simulink model "dev_RigTestWithNetwork"  (R2020b)
settings: Solver=VariableStepAuto  StartTime=0.0  StopTime=800  RelTol=1e-3
model workspace (MAT data in the model file):
  G_sup_tsp = Simulink.Signal
  G_sup_tsp.DataType = 'double'
  G_sup_tsp.Dimensions = -1
  G_sup_tsp.DimensionsMode = 'auto'
  G_sup_tsp.Complexity = 'real'
  G_sup_tsp.SampleTime = -1
  G_sup_tsp.SamplingMode = 'auto'
  G_sup_tsp.InitialValue = '175'
undefined symbols (not defined in the file): WLAN
libraries: truetime x9, IMT_Library x8, simulink_extras x4, slpidlib x2
settings Model: Creator=Mr_Li  LastModifiedBy=Mr_Li

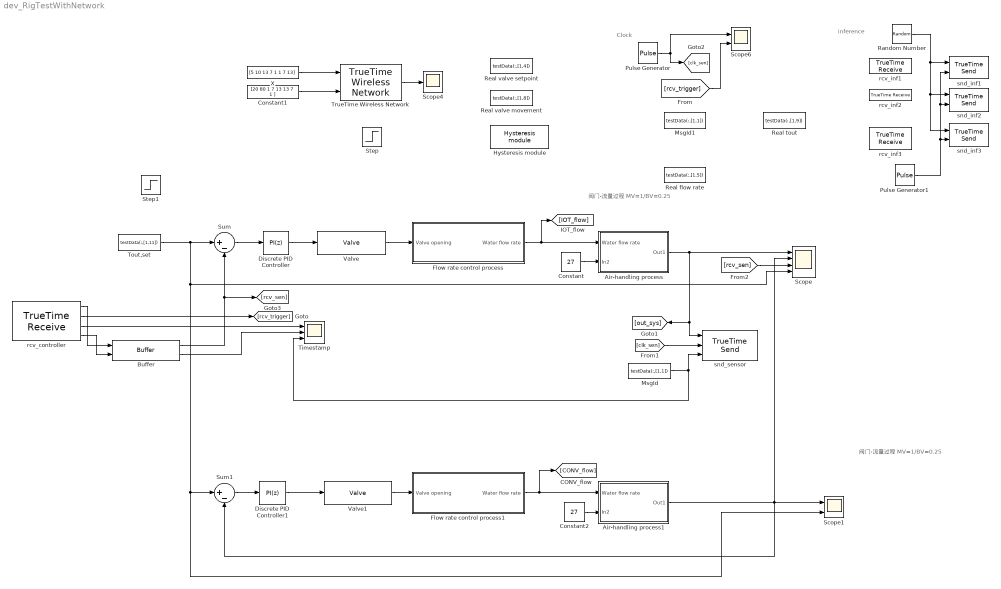
== system dev_RigTestWithNetwork ==
  note: inference
  note: 阀门-流量过程
      | MV=1/BV=0.25
  note: Clock
  note: 阀门-流量过程
      | MV=1/BV=0.25
  Air-handling process : Subsystem
  Air-handling process1 : Subsystem
  Buffer : IMT_Library/Buffer  initId=0  initValue=26
      settings: SourceProductName=Imitation
  Constant : Constant  Value=27
  Constant1 : Constant  Value=[20 80 1 7 13 13 7 1 ]  VectorParams1D=off
  Constant2 : Constant  Value=27
  Discrete PID Controller : slpidlib/PID Controller  Controller=PI  Form=Parallel  TimeDomain=Discrete-time  UseExternalTs=off  SampleTime=1  IntegratorMethod=Forward Euler  FilterMethod=Forward Euler  ControllerParametersSource=internal  P=0.5  I=0.0075  D=0  UseFilter=on  N=100  TunerSelectOption=Frequency Response Based  InitialConditionSource=internal  InitialConditionForIntegrator=0  InitialConditionForFilter=0  DifferentiatorICPrevScaledInput=0  ExternalReset=none  TrackingMode=off  Kt=1  LimitOutput=off  SatLimitsSource=internal  UpperSaturationLimit=inf  LowerSaturationLimit=-inf  LinearizeAsGain=off  AntiWindupMode=none  Kb=1  POutMin=[]  POutMax=[]  IOutMin=[]  IOutMax=[]  DOutMin=[]  DOutMax=[]  NOutMin=[]  NOutMax=[]  SumOutMin=[]  SumOutMax=[]  SaturationOutMin=[]  SaturationOutMax=[]  PParamMin=[]  PParamMax=[]  IParamMin=[]  IParamMax=[]  DParamMin=[]  DParamMax=[]  NParamMin=[]  NParamMax=[]  KbParamMin=[]  KbParamMax=[]  KtParamMin=[]  KtParamMax=[]  KbOutMin=[]  KbOutMax=[]  KtOutMin=[]  KtOutMax=[]  IntegratorOutMin=[]  IntegratorOutMax=[]  FilterOutMin=[]  FilterOutMax=[]  SumI1OutMin=[]  SumI1OutMax=[]  SumI2OutMin=[]  SumI2OutMax=[]  SumI3OutMin=[]  SumI3OutMax=[]  SumI4OutMin=[]  SumI4OutMax=[]  SumDOutMin=[]  SumDOutMax=[]  DifferentiatorOutMin=[]  DifferentiatorOutMax=[]  FilterDiffOutCoefMin=[]  FilterDiffOutCoefMax=[]  ReciprocalOutMin=[]  ReciprocalOutMax=[]  SumDenOutMin=[]  SumDenOutMax=[]  SumNumOutMin=[]  SumNumOutMax=[]  DivideOutMin=[]  DivideOutMax=[]  UdiffTsProdOutMin=[]  UdiffTsProdOutMax=[]  NTsProdOutMin=[]  NTsProdOutMax=[]  UintegralTsProdOutMin=[]  UintegralTsProdOutMax=[]  UngainTsProdOutMin=[]  UngainTsProdOutMax=[]  IntegratorContinuousStateAttributes=''  IntegratorStateMustResolveToSignalObject=off  IntegratorRTWStateStorageClass=Auto  FilterContinuousStateAttributes=''  FilterStateMustResolveToSignalObject=off  FilterRTWStateStorageClass=Auto  ParallelPVariant=InternalParameters  IdealPVariant=Disabled  IVariant=InternalParameters  DVariant=Disabled  IntegratorVariant=Discrete  SatVariant=Disabled  AWVariant=Passthrough  PCopyVariant=Disabled  TRVariant=Disabled  FdbkBlocksVariant=Forward  IdealPFdbkVariant=Disabled  SatFdbkVariant=Disabled  DerivativeFilterVariant=Disabled  NVariant=Disabled  NCopyVariant=Disabled_SignalSpec  FilterICVariant=Disabled  IntegratorICVariant=InternalICs  ExternalResetVariant=Disabled  TRSumVariant=Passthrough  SumFdbkVariant=Disabled  SumVariant=Sum_PI  TsampFilterVariant=InternalTs  TsampNgainVariant=Passthrough  TsampIntegralVariant=Passthrough  ExternalSaturationOutDataTypeStr=Inherit: Same as second input
  Discrete PID Controller1 : slpidlib/PID Controller  Controller=PI  Form=Parallel  TimeDomain=Discrete-time  UseExternalTs=off  SampleTime=1  IntegratorMethod=Forward Euler  FilterMethod=Forward Euler  ControllerParametersSource=internal  P=0.5  I=0.0075  D=0  UseFilter=on  N=100  TunerSelectOption=Frequency Response Based  InitialConditionSource=internal  InitialConditionForIntegrator=0  InitialConditionForFilter=0  DifferentiatorICPrevScaledInput=0  ExternalReset=none  TrackingMode=off  Kt=1  LimitOutput=off  SatLimitsSource=internal  UpperSaturationLimit=inf  LowerSaturationLimit=-inf  LinearizeAsGain=off  AntiWindupMode=none  Kb=1  POutMin=[]  POutMax=[]  IOutMin=[]  IOutMax=[]  DOutMin=[]  DOutMax=[]  NOutMin=[]  NOutMax=[]  SumOutMin=[]  SumOutMax=[]  SaturationOutMin=[]  SaturationOutMax=[]  PParamMin=[]  PParamMax=[]  IParamMin=[]  IParamMax=[]  DParamMin=[]  DParamMax=[]  NParamMin=[]  NParamMax=[]  KbParamMin=[]  KbParamMax=[]  KtParamMin=[]  KtParamMax=[]  KbOutMin=[]  KbOutMax=[]  KtOutMin=[]  KtOutMax=[]  IntegratorOutMin=[]  IntegratorOutMax=[]  FilterOutMin=[]  FilterOutMax=[]  SumI1OutMin=[]  SumI1OutMax=[]  SumI2OutMin=[]  SumI2OutMax=[]  SumI3OutMin=[]  SumI3OutMax=[]  SumI4OutMin=[]  SumI4OutMax=[]  SumDOutMin=[]  SumDOutMax=[]  DifferentiatorOutMin=[]  DifferentiatorOutMax=[]  FilterDiffOutCoefMin=[]  FilterDiffOutCoefMax=[]  ReciprocalOutMin=[]  ReciprocalOutMax=[]  SumDenOutMin=[]  SumDenOutMax=[]  SumNumOutMin=[]  SumNumOutMax=[]  DivideOutMin=[]  DivideOutMax=[]  UdiffTsProdOutMin=[]  UdiffTsProdOutMax=[]  NTsProdOutMin=[]  NTsProdOutMax=[]  UintegralTsProdOutMin=[]  UintegralTsProdOutMax=[]  UngainTsProdOutMin=[]  UngainTsProdOutMax=[]  IntegratorContinuousStateAttributes=''  IntegratorStateMustResolveToSignalObject=off  IntegratorRTWStateStorageClass=Auto  FilterContinuousStateAttributes=''  FilterStateMustResolveToSignalObject=off  FilterRTWStateStorageClass=Auto  ParallelPVariant=InternalParameters  IdealPVariant=Disabled  IVariant=InternalParameters  DVariant=Disabled  IntegratorVariant=Discrete  SatVariant=Disabled  AWVariant=Passthrough  PCopyVariant=Disabled  TRVariant=Disabled  FdbkBlocksVariant=Forward  IdealPFdbkVariant=Disabled  SatFdbkVariant=Disabled  DerivativeFilterVariant=Disabled  NVariant=Disabled  NCopyVariant=Disabled_SignalSpec  FilterICVariant=Disabled  IntegratorICVariant=InternalICs  ExternalResetVariant=Disabled  TRSumVariant=Passthrough  SumFdbkVariant=Disabled  SumVariant=Sum_PI  TsampFilterVariant=InternalTs  TsampNgainVariant=Passthrough  TsampIntegralVariant=Passthrough  ExternalSaturationOutDataTypeStr=Inherit: Same as second input
  Flow rate control process : Subsystem
  Flow rate control process1 : Subsystem
  Hysteresis module : IMT_Library/Hysteresis module  hysteresisSize=4.5
      settings: SourceProductName=Imitation
  MsgId : FromWorkspace  VariableName=testData(:,[1,1])  SampleTime=1
  MsgId1 : FromWorkspace  VariableName=testData(:,[1,1])  SampleTime=1
  Pulse Generator : DiscretePulseGenerator  SampleTime=0.5
  Pulse Generator1 : DiscretePulseGenerator
  Random Number : RandomNumber  SampleTime=1
  Real flow rate : FromWorkspace  VariableName=testData(:,[1,5])
  Real tout : FromWorkspace  VariableName=testData(:,[1,9])
  Real valve movement : FromWorkspace  VariableName=testData(:,[1,8])  SampleTime=1
  Real valve setpoint : FromWorkspace  VariableName=testData(:,[1,4])  SampleTime=1
  Scope : Scope  NumInputPorts=4
  Scope1 : Scope  NumInputPorts=2
  Scope4 : Scope
  Scope6 : Scope  NumInputPorts=2
  Step : Step  Time=18  After=0.31  SampleTime=0
  Step1 : Step  After=45  SampleTime=0
  Sum : Sum  Inputs=|+-
  Sum1 : Sum  Inputs=|+-
  Timestamp : Scope  NumInputPorts=3
  Tout,set : FromWorkspace  VariableName=testData(:,[1,11])  SampleTime=1
  TrueTime Wireless Network : truetime/TrueTime Wireless  Network  nwtype=802.11b (WLAN)  nwnbr=1  nnodes=8  rate=800000  minsize=272  transpower=30  threshold=-48  use_pathloss_function=default  pathloss=4.0  acktimeout=1  retrylimit=3  error_threshold=0.04  lossprob=0.4  seed=0  scheduleoutput=on  poweroutput=off
  Valve : IMT_Library/Valve  upper=101  lower=1.2  movementThreshold=1
      settings: SourceProductName=Imitation
  Valve1 : IMT_Library/Valve  upper=101  lower=1.2  movementThreshold=1
      settings: SourceProductName=Imitation
  X : Constant  Value="[5 10 13 7 1  1 7 13]"  VectorParams1D=off
  rcv_controller : truetime/TrueTime Receive  nwnbr=1  receiver=2  outdim=1  triggeroutput=on  senderoutput=off  lengthoutput=off  priorityoutput=off  timestampoutput=on  signalpoweroutput=off  msgIDoutput=on
  rcv_inf1 : truetime/TrueTime Receive  nwnbr=1  receiver=4  outdim=1  triggeroutput=off  senderoutput=off  lengthoutput=off  priorityoutput=off  timestampoutput=off  signalpoweroutput=off  msgIDoutput=off
  rcv_inf2 : truetime/TrueTime Receive  nwnbr=1  receiver=6  outdim=1  triggeroutput=off  senderoutput=off  lengthoutput=off  priorityoutput=off  timestampoutput=off  signalpoweroutput=off  msgIDoutput=off
  rcv_inf3 : truetime/TrueTime Receive  nwnbr=1  receiver=8  outdim=1  triggeroutput=on  senderoutput=off  lengthoutput=off  priorityoutput=off  timestampoutput=off  signalpoweroutput=off  msgIDoutput=off
  snd_inf1 : truetime/TrueTime Send  trigger=falling  nwnbr=1  sender=3  indim=1  recsource=internal  receiver=4  lengthsource=internal  length=1000  priosource=internal  prio=1  msgIDsource=internal  msgID=0  dynamicSegment=dynamic
  snd_inf2 : truetime/TrueTime Send  trigger=falling  nwnbr=1  sender=5  indim=1  recsource=internal  receiver=6  lengthsource=internal  length=1000  priosource=internal  prio=1  msgIDsource=internal  msgID=0  dynamicSegment=dynamic
  snd_inf3 : truetime/TrueTime Send  trigger=falling  nwnbr=1  sender=7  indim=1  recsource=internal  receiver=8  lengthsource=internal  length=1000  priosource=internal  prio=1  msgIDsource=internal  msgID=0  dynamicSegment=dynamic
  snd_sensor : truetime/TrueTime Send  trigger=falling  nwnbr=1  sender=1  indim=1  recsource=internal  receiver=2  lengthsource=internal  length=1000  priosource=internal  prio=1  msgIDsource=external  msgID=0  dynamicSegment=dynamic
  wires:
  Sum/1 -> Discrete PID Controller/1
  Discrete PID Controller/1 -> Valve/1
  X/1 -> TrueTime Wireless Network/1
  Constant1/1 -> TrueTime Wireless Network/2
  TrueTime Wireless Network/1 -> Scope4/1
  rcv_controller/2 -> [rcv_trigger]
  rcv_controller/1 -> Buffer/1
  Buffer/1 -> [rcv_sen], Sum/2
  [clk_sen] -> snd_sensor/2
  Pulse Generator/1 -> Scope6/1, [clk_sen]
  Air-handling process1/1(Out1) -> Scope/2, Scope1/1, Sum1/2
  Sum1/1 -> Discrete PID Controller1/1
  Flow rate control process1/1(Water flow rate) -> Air-handling process1/1(Water flow rate), [CONV_flow]
  rcv_controller/3 -> Timestamp/1
  MsgId/1 -> snd_sensor/3, Timestamp/3
  Pulse Generator1/1 -> snd_inf1/2, snd_inf2/2, snd_inf3/2
  Random Number/1 -> snd_inf3/1, snd_inf2/1, snd_inf1/1
  [rcv_sen] -> Scope/3
  [rcv_trigger] -> Scope6/2
  Tout,set/1 -> Scope1/2, Sum1/1, Scope/4, Sum/1
  Valve1/1 -> Flow rate control process1/1(Valve opening)
  Discrete PID Controller1/1 -> Valve1/1
  Flow rate control process/1(Water flow rate) -> [IOT_flow], Air-handling process/1(Water flow rate)
  Valve/1 -> Flow rate control process/1(Valve opening)
  Air-handling process/1(Out1) -> Scope/1, snd_sensor/1, [out_sys]
  Constant/1 -> Air-handling process/2(In2)
  Constant2/1 -> Air-handling process1/2(In2)
  rcv_controller/4 -> Buffer/2
  Buffer/2 -> Timestamp/2

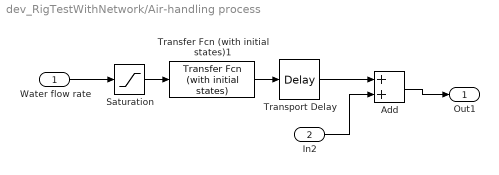
== system dev_RigTestWithNetwork/Air-handling process ==
  Water flow rate : Inport
  In2 : Inport  Port=2
  Add : Sum
  Saturation : Saturate  UpperLimit=0.25  LowerLimit=0
  Transfer Fcn (with initial states)1 : simulink_extras/Additional Linear/Transfer Fcn (with initial states)  N=[105]  D=[380 40 1]  X0=0
  Transport Delay : TransportDelay  DelayTime=0
  Out1 : Outport
  wires:
  Transfer Fcn (with initial states)1/1 -> Transport Delay/1
  Add/1 -> Out1/1
  Water flow rate/1 -> Saturation/1
  In2/1 -> Add/2
  Saturation/1 -> Transfer Fcn (with initial states)1/1
  Transport Delay/1 -> Add/1

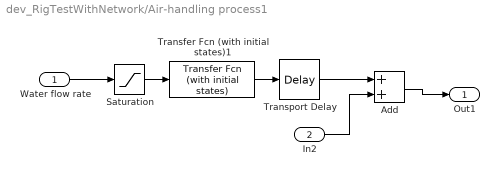
== system dev_RigTestWithNetwork/Air-handling process1 ==
  Water flow rate : Inport
  In2 : Inport  Port=2
  Add : Sum
  Saturation : Saturate  UpperLimit=0.25  LowerLimit=0
  Transfer Fcn (with initial states)1 : simulink_extras/Additional Linear/Transfer Fcn (with initial states)  N=[105]  D=[380 40 1]  X0=0
  Transport Delay : TransportDelay  DelayTime=0
  Out1 : Outport
  wires:
  Transfer Fcn (with initial states)1/1 -> Transport Delay/1
  Add/1 -> Out1/1
  Water flow rate/1 -> Saturation/1
  In2/1 -> Add/2
  Saturation/1 -> Transfer Fcn (with initial states)1/1
  Transport Delay/1 -> Add/1

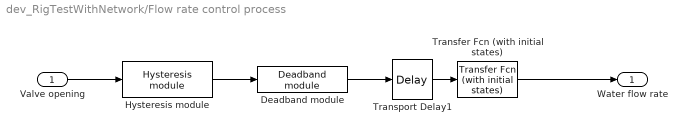
== system dev_RigTestWithNetwork/Flow rate control process ==
  Valve opening : Inport
  Deadband module : IMT_Library/Deadband module  upper=22.5  lower=6.5
      settings: SourceProductName=Imitation
  Hysteresis module : IMT_Library/Hysteresis module  hysteresisSize=4.5
      settings: SourceProductName=Imitation
  Transfer Fcn (with initial states) : simulink_extras/Additional Linear/Transfer Fcn (with initial states)  N=[0.032]  D=[3.6 1]  X0=0
  Transport Delay1 : TransportDelay  DelayTime=3
  Water flow rate : Outport
  wires:
  Valve opening/1 -> Hysteresis module/1
  Deadband module/1 -> Transport Delay1/1
  Transfer Fcn (with initial states)/1 -> Water flow rate/1
  Transport Delay1/1 -> Transfer Fcn (with initial states)/1
  Hysteresis module/1 -> Deadband module/1

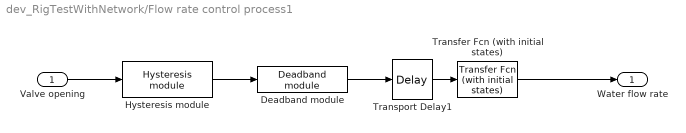
== system dev_RigTestWithNetwork/Flow rate control process1 ==
  Valve opening : Inport
  Deadband module : IMT_Library/Deadband module  upper=22.5  lower=6.5
      settings: SourceProductName=Imitation
  Hysteresis module : IMT_Library/Hysteresis module  hysteresisSize=4.5
      settings: SourceProductName=Imitation
  Transfer Fcn (with initial states) : simulink_extras/Additional Linear/Transfer Fcn (with initial states)  N=[0.032]  D=[3.6 1]  X0=0
  Transport Delay1 : TransportDelay  DelayTime=3
  Water flow rate : Outport
  wires:
  Valve opening/1 -> Hysteresis module/1
  Deadband module/1 -> Transport Delay1/1
  Transfer Fcn (with initial states)/1 -> Water flow rate/1
  Transport Delay1/1 -> Transfer Fcn (with initial states)/1
  Hysteresis module/1 -> Deadband module/1
